simulink model "sampleModel646original"  (R2021b)
settings: Solver=VariableStepAuto  StartTime=0.0  StopTime=10.0  RelTol=1e-3
undefined symbols (not defined in the file): DiscIntNeverNeededParam, Newton, Raphson, sigbuilder_block
libraries: simulink x194, slpidlib x27
(part 5 of 5)

== system sampleModel646original/emi_506 ==
  In1 : Inport
  emi_507 : Inport  Port=2
  emi_509 : Relay
  emi_{510..511,514,519,521,523} (6 alike) : simulink/Discrete/Transfer Fcn First Order  PoleZ=0.95  ICPrevOutput=0.0  DoSatur=off
  emi_512 : Sum  Inputs=+
  emi_513 : DiscreteIntegrator  SampleTime=-1  ICPrevOutput=DiscIntNeverNeededParam  ICPrevScaledInput=DiscIntNeverNeededParam
  emi_515 : DiscreteIntegrator  SampleTime=-1  ICPrevOutput=DiscIntNeverNeededParam  ICPrevScaledInput=DiscIntNeverNeededParam
  emi_516 : DiscreteFir
  emi_517 : Abs
  emi_518 : simulink/Discrete/Difference  ICPrevInput=0.0  OutMin=[]  OutMax=[]  OutDataType=fixdt(1, 16)  OutScaling=2^-10  DoSatur=off
  emi_520 : MinMax
  emi_522 : DiscreteZeroPole  Poles=[0 0.5]  Gain=1  SampleTime=-1
  emi_524 : simulink/Discrete/Discrete Derivative  gainval=1.0  ICPrevScaledInput=0.0  OutMin=[]  OutMax=[]  OutDataType=fixdt(1, 16)  OutScaling=2^-10  DoSatur=off
  emi_525 : simulink/Discrete/Difference  ICPrevInput=0.0  OutMin=[]  OutMax=[]  OutDataType=fixdt(1, 16)  OutScaling=2^-10  DoSatur=off
  emi_526 : Product  Inputs=*
  emi_527 : Math  SaturateOnIntegerOverflow=on
  emi_528 : simulink/Discontinuities/Rate Limiter Dynamic
  emi_529 : Clock
  Out1 : Outport
  emi_508 : Outport  Port=2
  wires:
  In1/1 -> Out1/1
  emi_509/1 -> emi_510/1
  emi_510/1 -> emi_511/1
  emi_511/1 -> emi_512/1
  emi_512/1 -> emi_513/1
  emi_513/1 -> emi_514/1
  emi_514/1 -> emi_515/1
  emi_515/1 -> emi_516/1
  emi_516/1 -> emi_517/1
  emi_517/1 -> emi_518/1
  emi_518/1 -> emi_519/1
  emi_519/1 -> emi_520/1
  emi_520/1 -> emi_521/1
  emi_521/1 -> emi_522/1
  emi_522/1 -> emi_523/1
  emi_523/1 -> emi_524/1
  emi_524/1 -> emi_525/1
  emi_525/1 -> emi_526/1
  emi_526/1 -> emi_527/1
  emi_527/1 -> emi_528/1
  emi_529/1 -> emi_509/1
  emi_528/1 -> emi_508/1

== system sampleModel646original/emi_536 ==
  emi_543 : Inport
  Action Port : ActionPort  ActionPortLabel=if(0 > u1)
  emi_540 : Abs
  emi_{541..542,549..550} (4 alike) : MinMax
  emi_545 : Trigonometry
  emi_546 : Trigonometry
  emi_547 : UnaryMinus
  emi_548 : Sin  TimeSource=Use external signal  SampleTime=0
  emi_551 : Sum  Inputs=+
  emi_552 : Sin  TimeSource=Use external signal  SampleTime=0
  emi_553 : Sqrt  Operator=rSqrt  SaturateOnIntegerOverflow=on
  emi_554 : Ground
  emi_544 : Outport
  wires:
  emi_543/1 -> emi_540/1
  emi_540/1 -> emi_541/1
  emi_541/1 -> emi_542/1
  emi_545/1 -> emi_546/1
  emi_546/1 -> emi_547/1
  emi_547/1 -> emi_548/1
  emi_548/1 -> emi_549/1
  emi_549/1 -> emi_550/1
  emi_550/1 -> emi_551/1
  emi_551/1 -> emi_552/1
  emi_552/1 -> emi_553/1
  emi_554/1 -> emi_545/1
  emi_553/1 -> emi_544/1

== system sampleModel646original/emi_557 ==
  In1 : Inport
  emi_558 : Inport  Port=2
  emi_560 : Gain
  emi_561 : simulink/Discrete/Discrete Derivative  gainval=1.0  ICPrevScaledInput=0.0  OutMin=[]  OutMax=[]  OutDataType=fixdt(1, 16)  OutScaling=2^-10  DoSatur=off
  emi_562 : DiscreteIntegrator  SampleTime=-1  ICPrevOutput=DiscIntNeverNeededParam  ICPrevScaledInput=DiscIntNeverNeededParam
  emi_563 : RateLimiter  SampleTimeMode=inherited
  emi_564 : Product  Inputs=*
  emi_565 : MinMax
  emi_566 : DiscreteTransferFcn
  emi_567 : simulink/Discontinuities/PWM  DisableCoverage=on  Period=1  DisallowZeroDutyCycle=off  RunAtFixedTimeIntervals=off  SampleTime=0.1
  emi_568 : Gain
  emi_569 : Abs
  emi_570 : Trigonometry
  emi_571 : Sqrt  Operator=rSqrt  SaturateOnIntegerOverflow=on
  emi_572 : Sum  Inputs=+
  emi_573 : simulink/Sources/Chirp Signal  f1=0.1  T=100  f2=1
  Out1 : Outport
  emi_559 : Outport  Port=2
  wires:
  In1/1 -> Out1/1
  emi_560/1 -> emi_561/1
  emi_561/1 -> emi_562/1
  emi_562/1 -> emi_563/1
  emi_563/1 -> emi_564/1
  emi_564/1 -> emi_565/1
  emi_565/1 -> emi_566/1
  emi_566/1 -> emi_567/1
  emi_567/1 -> emi_568/1
  emi_568/1 -> emi_569/1
  emi_569/1 -> emi_570/1
  emi_570/1 -> emi_571/1
  emi_571/1 -> emi_572/1
  emi_573/1 -> emi_560/1
  emi_572/1 -> emi_559/1

== system sampleModel646original/emi_580 ==
  emi_587 : Inport
  Action Port : ActionPort  ActionPortLabel=if(0 > u1)
  emi_{584,586,589,594} (4 alike) : Abs
  emi_585 : Math  SaturateOnIntegerOverflow=on
  emi_590 : Gain
  emi_591 : Sqrt  Operator=rSqrt  SaturateOnIntegerOverflow=on
  emi_592 : Gain
  emi_593 : Rounding
  emi_595 : Trigonometry
  emi_596 : Product  Inputs=*
  emi_597 : Sum  Inputs=+
  emi_598 : Rounding
  emi_599 : Sin  TimeSource=Use external signal  SampleTime=0
  emi_600 : Sqrt  Operator=rSqrt  SaturateOnIntegerOverflow=on
  emi_601 : Trigonometry
  emi_602 : Ground
  emi_588 : Outport
  wires:
  emi_587/1 -> emi_584/1
  emi_584/1 -> emi_585/1
  emi_585/1 -> emi_586/1
  emi_589/1 -> emi_590/1
  emi_590/1 -> emi_591/1
  emi_591/1 -> emi_592/1
  emi_592/1 -> emi_593/1
  emi_593/1 -> emi_594/1
  emi_594/1 -> emi_595/1
  emi_595/1 -> emi_596/1
  emi_596/1 -> emi_597/1
  emi_597/1 -> emi_598/1
  emi_598/1 -> emi_599/1
  emi_599/1 -> emi_600/1
  emi_600/1 -> emi_601/1
  emi_602/1 -> emi_589/1
  emi_601/1 -> emi_588/1

== system sampleModel646original/emi_605 ==
  In1 : Inport
  emi_606 : Inport  Port=2
  emi_608 : simulink/Discontinuities/Wrap To Zero  Threshold=255
      settings: SourceProductBaseCode=SL
  emi_609 : simulink/Discontinuities/Rate Limiter Dynamic
  emi_610 : DiscreteTransferFcn
  emi_611 : RateLimiter  SampleTimeMode=inherited
  emi_612 : Gain
  emi_613 : simulink/Discrete/Transfer Fcn First Order  PoleZ=0.95  ICPrevOutput=0.0  DoSatur=off
  emi_614 : simulink/Discontinuities/Saturation Dynamic  OutMin=[]  OutMax=[]  OutDataTypeStr=Inherit: Same as second input  OutDataType=fixdt(1, 16)  OutScaling=2^-10  DoSatur=off
  emi_615 : Sqrt  Operator=rSqrt  SaturateOnIntegerOverflow=on
  emi_616 : Sqrt  Operator=rSqrt  SaturateOnIntegerOverflow=on
  emi_617 : Sin  TimeSource=Use external signal  SampleTime=0
  emi_618 : Clock
  Out1 : Outport
  emi_607 : Outport  Port=2
  wires:
  In1/1 -> Out1/1
  emi_608/1 -> emi_609/1
  emi_609/1 -> emi_610/1
  emi_610/1 -> emi_611/1
  emi_611/1 -> emi_612/1
  emi_612/1 -> emi_613/1
  emi_613/1 -> emi_614/1
  emi_614/1 -> emi_615/1
  emi_615/1 -> emi_616/1
  emi_616/1 -> emi_617/1
  emi_618/1 -> emi_608/1
  emi_617/1 -> emi_607/1

== system sampleModel646original/emi_61 ==
  emi_68 : Inport
  Action Port : ActionPort  ActionPortLabel=if(0 > u1)
  emi_65 : MinMax  SampleTime=1
  emi_66 : MinMax  SampleTime=1
  emi_67 : Math  SampleTime=1  SaturateOnIntegerOverflow=on
  emi_70 : Gain
  emi_71 : UnaryMinus
  emi_72 : Abs
  emi_73 : Gain
  emi_74 : Ground
  emi_69 : Outport
  wires:
  emi_68/1 -> emi_65/1
  emi_65/1 -> emi_66/1
  emi_66/1 -> emi_67/1
  emi_70/1 -> emi_71/1
  emi_71/1 -> emi_72/1
  emi_72/1 -> emi_73/1
  emi_74/1 -> emi_70/1
  emi_73/1 -> emi_69/1

== system sampleModel646original/emi_625 ==
  emi_632 : Inport
  Action Port : ActionPort  ActionPortLabel=if(0 > u1)
  emi_629 : Abs
  emi_{630..631,643,647,649,651} (6 alike) : MinMax
  emi_634 : Product  Inputs=*
  emi_635 : Trigonometry
  emi_636 : Product  Inputs=*
  emi_637 : Sqrt  Operator=rSqrt  SaturateOnIntegerOverflow=on
  emi_638 : UnaryMinus
  emi_639 : Rounding
  emi_640 : Sin  TimeSource=Use external signal  SampleTime=0
  emi_641 : Trigonometry
  emi_642 : Product  Inputs=*
  emi_644 : Trigonometry
  emi_645 : UnaryMinus
  emi_646 : Sin  TimeSource=Use external signal  SampleTime=0
  emi_648 : Gain
  emi_650 : Abs
  emi_652 : Ground
  emi_633 : Outport
  wires:
  emi_632/1 -> emi_629/1
  emi_629/1 -> emi_630/1
  emi_630/1 -> emi_631/1
  emi_634/1 -> emi_635/1
  emi_635/1 -> emi_636/1
  emi_636/1 -> emi_637/1
  emi_637/1 -> emi_638/1
  emi_638/1 -> emi_639/1
  emi_639/1 -> emi_640/1
  emi_640/1 -> emi_641/1
  emi_641/1 -> emi_642/1
  emi_642/1 -> emi_643/1
  emi_643/1 -> emi_644/1
  emi_644/1 -> emi_645/1
  emi_645/1 -> emi_646/1
  emi_646/1 -> emi_647/1
  emi_647/1 -> emi_648/1
  emi_648/1 -> emi_649/1
  emi_649/1 -> emi_650/1
  emi_650/1 -> emi_651/1
  emi_652/1 -> emi_634/1
  emi_651/1 -> emi_633/1

== system sampleModel646original/emi_655 ==
  In1 : Inport
  emi_656 : Inport  Port=2
  emi_658 : Gain
  emi_659 : simulink/Discontinuities/Saturation Dynamic  OutMin=[]  OutMax=[]  OutDataTypeStr=Inherit: Same as second input  OutDataType=fixdt(1, 16)  OutScaling=2^-10  DoSatur=off
  emi_660 : simulink/Discrete/Transfer Fcn First Order  PoleZ=0.95  ICPrevOutput=0.0  DoSatur=off
  emi_661 : Product  Inputs=*
  emi_662 : Relay
  emi_663 : simulink/Discontinuities/Rate Limiter Dynamic
  emi_664 : Sin  TimeSource=Use external signal  SampleTime=0
  emi_665 : DeadZone  SaturateOnIntegerOverflow=on
  emi_666 : DiscreteIntegrator  SampleTime=-1  ICPrevOutput=DiscIntNeverNeededParam  ICPrevScaledInput=DiscIntNeverNeededParam
  emi_667 : Quantizer
  emi_668 : simulink/Discontinuities/Saturation Dynamic  OutMin=[]  OutMax=[]  OutDataTypeStr=Inherit: Same as second input  OutDataType=fixdt(1, 16)  OutScaling=2^-10  DoSatur=off
  emi_669 : UnaryMinus
  emi_670 : VariablePulseGenerator  SampleTime=0.1
  emi_671 : simulink/Discontinuities/Saturation Dynamic  OutMin=[]  OutMax=[]  OutDataTypeStr=Inherit: Same as second input  OutDataType=fixdt(1, 16)  OutScaling=2^-10  DoSatur=off
  emi_672 : simulink/Discrete/Transfer Fcn First Order  PoleZ=0.95  ICPrevOutput=0.0  DoSatur=off
  emi_673 : Abs
  emi_674 : RateLimiter  SampleTimeMode=inherited
  emi_675 : Abs
  emi_676 : Gain
  emi_677 : Rounding
  emi_678 : DiscreteTransferFcn
  emi_679 : VariablePulseGenerator  SampleTime=0.1
  emi_680 : Product  Inputs=*
  emi_681 : simulink/Discontinuities/Wrap To Zero  Threshold=255
      settings: SourceProductBaseCode=SL
  emi_682 : RateLimiter  SampleTimeMode=inherited
  emi_683 : Quantizer
  emi_684 : Relay
  emi_685 : simulink/Discrete/Discrete Derivative  gainval=1.0  ICPrevScaledInput=0.0  OutMin=[]  OutMax=[]  OutDataType=fixdt(1, 16)  OutScaling=2^-10  DoSatur=off
  emi_686 : simulink/Discrete/Transfer Fcn First Order  PoleZ=0.95  ICPrevOutput=0.0  DoSatur=off
  emi_687 : Math  SaturateOnIntegerOverflow=on
  emi_688 : MinMax
  emi_689 : simulink/Sources/Repeating Sequence Interpolated  OutValues=[3 1 4 2 1].'  TimeValues=[0 0.1 0.5 0.6 1].'  LookUpMeth=Interpolation-Use End Values  tsamp=0.01  OutMin=[]  OutMax=[]  OutDataTypeStr=double  OutputDataTypeScalingMode=double  OutDataType=fixdt(0,8)  OutScaling=2^-10
  Out1 : Outport
  emi_657 : Outport  Port=2
  wires:
  In1/1 -> Out1/1
  emi_658/1 -> emi_659/1
  emi_659/1 -> emi_660/1
  emi_660/1 -> emi_661/1
  emi_661/1 -> emi_662/1
  emi_662/1 -> emi_663/1
  emi_663/1 -> emi_664/1
  emi_664/1 -> emi_665/1
  emi_665/1 -> emi_666/1
  emi_666/1 -> emi_667/1
  emi_667/1 -> emi_668/1
  emi_668/1 -> emi_669/1
  emi_669/1 -> emi_670/1
  emi_670/1 -> emi_671/1
  emi_671/1 -> emi_672/1
  emi_672/1 -> emi_673/1
  emi_673/1 -> emi_674/1
  emi_674/1 -> emi_675/1
  emi_675/1 -> emi_676/1
  emi_676/1 -> emi_677/1
  emi_677/1 -> emi_678/1
  emi_678/1 -> emi_679/1
  emi_679/1 -> emi_680/1
  emi_680/1 -> emi_681/1
  emi_681/1 -> emi_682/1
  emi_682/1 -> emi_683/1
  emi_683/1 -> emi_684/1
  emi_684/1 -> emi_685/1
  emi_685/1 -> emi_686/1
  emi_686/1 -> emi_687/1
  emi_687/1 -> emi_688/1
  emi_689/1 -> emi_658/1
  emi_688/1 -> emi_657/1

== system sampleModel646original/emi_697 ==
  emi_704 : Inport
  Action Port : ActionPort  ActionPortLabel=if(0 > u1)
  emi_701 : MinMax
  emi_702 : MinMax
  emi_703 : Gain
  emi_706 : Sin  TimeSource=Use external signal  SampleTime=0
  emi_707 : Trigonometry
  emi_708 : Math  SaturateOnIntegerOverflow=on
  emi_709 : Rounding
  emi_710 : Abs
  emi_711 : MinMax
  emi_712 : Rounding
  emi_713 : Sum  Inputs=+
  emi_714 : Abs
  emi_715 : Ground
  emi_705 : Outport
  wires:
  emi_704/1 -> emi_701/1
  emi_701/1 -> emi_702/1
  emi_702/1 -> emi_703/1
  emi_706/1 -> emi_707/1
  emi_707/1 -> emi_708/1
  emi_708/1 -> emi_709/1
  emi_709/1 -> emi_710/1
  emi_710/1 -> emi_711/1
  emi_711/1 -> emi_712/1
  emi_712/1 -> emi_713/1
  emi_713/1 -> emi_714/1
  emi_715/1 -> emi_706/1
  emi_714/1 -> emi_705/1

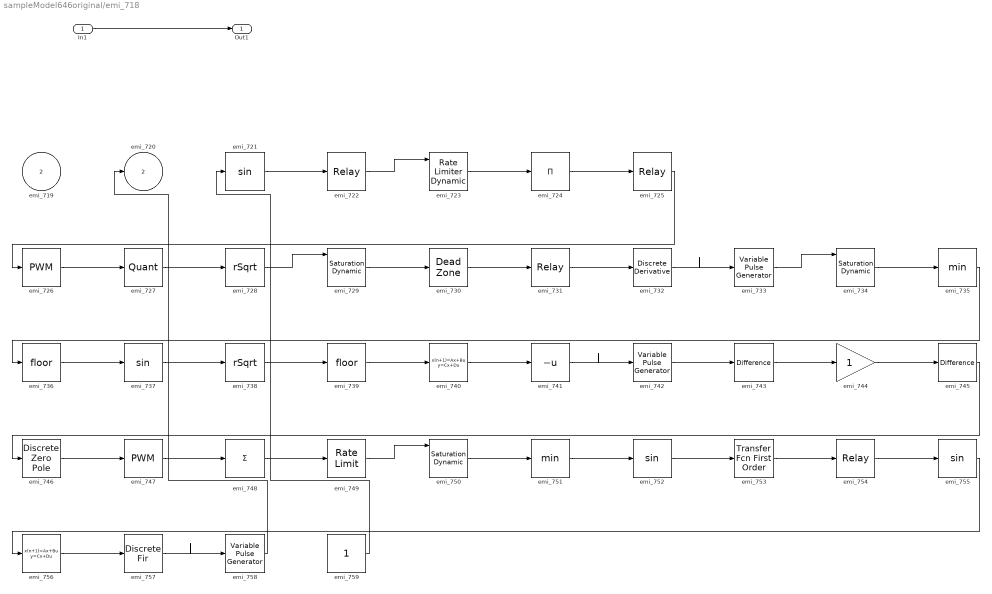
== system sampleModel646original/emi_718 ==
  In1 : Inport
  emi_719 : Inport  Port=2
  emi_{721,737,752,755} (4 alike) : Trigonometry
  emi_{722,725,731,754} (4 alike) : Relay
  emi_723 : simulink/Discontinuities/Rate Limiter Dynamic
  emi_724 : Product  Inputs=*
  emi_726 : simulink/Discontinuities/PWM  DisableCoverage=on  Period=1  DisallowZeroDutyCycle=off  RunAtFixedTimeIntervals=off  SampleTime=0.1
  emi_727 : Quantizer
  emi_728 : Sqrt  Operator=rSqrt  SaturateOnIntegerOverflow=on
  emi_729 : simulink/Discontinuities/Saturation Dynamic  OutMin=[]  OutMax=[]  OutDataTypeStr=Inherit: Same as second input  OutDataType=fixdt(1, 16)  OutScaling=2^-10  DoSatur=off
  emi_730 : DeadZone  SaturateOnIntegerOverflow=on
  emi_732 : simulink/Discrete/Discrete Derivative  gainval=1.0  ICPrevScaledInput=0.0  OutMin=[]  OutMax=[]  OutDataType=fixdt(1, 16)  OutScaling=2^-10  DoSatur=off
  emi_733 : VariablePulseGenerator  SampleTime=0.1
  emi_734 : simulink/Discontinuities/Saturation Dynamic  OutMin=[]  OutMax=[]  OutDataTypeStr=Inherit: Same as second input  OutDataType=fixdt(1, 16)  OutScaling=2^-10  DoSatur=off
  emi_735 : MinMax
  emi_736 : Rounding
  emi_738 : Sqrt  Operator=rSqrt  SaturateOnIntegerOverflow=on
  emi_739 : Rounding
  emi_740 : DiscreteStateSpace  SampleTime=-1
  emi_741 : UnaryMinus
  emi_742 : VariablePulseGenerator  SampleTime=0.1
  emi_743 : simulink/Discrete/Difference  ICPrevInput=0.0  OutMin=[]  OutMax=[]  OutDataType=fixdt(1, 16)  OutScaling=2^-10  DoSatur=off
  emi_744 : Gain
  emi_745 : simulink/Discrete/Difference  ICPrevInput=0.0  OutMin=[]  OutMax=[]  OutDataType=fixdt(1, 16)  OutScaling=2^-10  DoSatur=off
  emi_746 : DiscreteZeroPole  Poles=[0 0.5]  Gain=1  SampleTime=-1
  emi_747 : simulink/Discontinuities/PWM  DisableCoverage=on  Period=1  DisallowZeroDutyCycle=off  RunAtFixedTimeIntervals=off  SampleTime=0.1
  emi_748 : Sum  Inputs=+
  emi_749 : RateLimiter  SampleTimeMode=inherited
  emi_750 : simulink/Discontinuities/Saturation Dynamic  OutMin=[]  OutMax=[]  OutDataTypeStr=Inherit: Same as second input  OutDataType=fixdt(1, 16)  OutScaling=2^-10  DoSatur=off
  emi_751 : MinMax
  emi_753 : simulink/Discrete/Transfer Fcn First Order  PoleZ=0.95  ICPrevOutput=0.0  DoSatur=off
  emi_756 : DiscreteStateSpace  SampleTime=-1
  emi_757 : DiscreteFir
  emi_758 : VariablePulseGenerator  SampleTime=0.1
  emi_759 : Constant
  Out1 : Outport
  emi_720 : Outport  Port=2
  wires:
  In1/1 -> Out1/1
  emi_721/1 -> emi_722/1
  emi_722/1 -> emi_723/1
  emi_723/1 -> emi_724/1
  emi_724/1 -> emi_725/1
  emi_725/1 -> emi_726/1
  emi_726/1 -> emi_727/1
  emi_727/1 -> emi_728/1
  emi_728/1 -> emi_729/1
  emi_729/1 -> emi_730/1
  emi_730/1 -> emi_731/1
  emi_731/1 -> emi_732/1
  emi_732/1 -> emi_733/1
  emi_733/1 -> emi_734/1
  emi_734/1 -> emi_735/1
  emi_735/1 -> emi_736/1
  emi_736/1 -> emi_737/1
  emi_737/1 -> emi_738/1
  emi_738/1 -> emi_739/1
  emi_739/1 -> emi_740/1
  emi_740/1 -> emi_741/1
  emi_741/1 -> emi_742/1
  emi_742/1 -> emi_743/1
  emi_743/1 -> emi_744/1
  emi_744/1 -> emi_745/1
  emi_745/1 -> emi_746/1
  emi_746/1 -> emi_747/1
  emi_747/1 -> emi_748/1
  emi_748/1 -> emi_749/1
  emi_749/1 -> emi_750/1
  emi_750/1 -> emi_751/1
  emi_751/1 -> emi_752/1
  emi_752/1 -> emi_753/1
  emi_753/1 -> emi_754/1
  emi_754/1 -> emi_755/1
  emi_755/1 -> emi_756/1
  emi_756/1 -> emi_757/1
  emi_757/1 -> emi_758/1
  emi_759/1 -> emi_721/1
  emi_758/1 -> emi_720/1

== system sampleModel646original/emi_766 ==
  emi_773 : Inport
  Action Port : ActionPort  ActionPortLabel=if(0 > u1)
  emi_770 : MinMax
  emi_771 : Math  SaturateOnIntegerOverflow=on
  emi_772 : Math  SaturateOnIntegerOverflow=on
  emi_775 : Trigonometry
  emi_776 : Sum  Inputs=+
  emi_777 : Rounding
  emi_778 : Product  Inputs=*
  emi_779 : Trigonometry
  emi_780 : Sin  TimeSource=Use external signal  SampleTime=0
  emi_781 : Abs
  emi_782 : Sqrt  Operator=rSqrt  SaturateOnIntegerOverflow=on
  emi_783 : Sin  TimeSource=Use external signal  SampleTime=0
  emi_784 : Sqrt  Operator=rSqrt  SaturateOnIntegerOverflow=on
  emi_785 : Product  Inputs=*
  emi_786 : MinMax
  emi_787 : Abs
  emi_788 : Abs
  emi_{789,793,795..796} (4 alike) : Gain
  emi_790 : UnaryMinus
  emi_791 : MinMax
  emi_792 : Rounding
  emi_794 : Sqrt  Operator=rSqrt  SaturateOnIntegerOverflow=on
  emi_797 : Ground
  emi_774 : Outport
  wires:
  emi_773/1 -> emi_770/1
  emi_770/1 -> emi_771/1
  emi_771/1 -> emi_772/1
  emi_775/1 -> emi_776/1
  emi_776/1 -> emi_777/1
  emi_777/1 -> emi_778/1
  emi_778/1 -> emi_779/1
  emi_779/1 -> emi_780/1
  emi_780/1 -> emi_781/1
  emi_781/1 -> emi_782/1
  emi_782/1 -> emi_783/1
  emi_783/1 -> emi_784/1
  emi_784/1 -> emi_785/1
  emi_785/1 -> emi_786/1
  emi_786/1 -> emi_787/1
  emi_787/1 -> emi_788/1
  emi_788/1 -> emi_789/1
  emi_789/1 -> emi_790/1
  emi_790/1 -> emi_791/1
  emi_791/1 -> emi_792/1
  emi_792/1 -> emi_793/1
  emi_793/1 -> emi_794/1
  emi_794/1 -> emi_795/1
  emi_795/1 -> emi_796/1
  emi_797/1 -> emi_775/1
  emi_796/1 -> emi_774/1

== system sampleModel646original/emi_77 ==
  In1 : Inport
  emi_78 : Inport  Port=2
  emi_80 : DiscreteIntegrator  SampleTime=-1  ICPrevOutput=DiscIntNeverNeededParam  ICPrevScaledInput=DiscIntNeverNeededParam
  emi_81 : simulink/Discontinuities/Wrap To Zero  Threshold=255
      settings: SourceProductBaseCode=SL
  emi_82 : DigitalClock
  Out1 : Outport
  emi_79 : Outport  Port=2
  wires:
  In1/1 -> Out1/1
  emi_80/1 -> emi_81/1
  emi_82/1 -> emi_80/1
  emi_81/1 -> emi_79/1

== system sampleModel646original/emi_800 ==
  In1 : Inport
  emi_801 : Inport  Port=2
  emi_803 : simulink/Discrete/Transfer Fcn First Order  PoleZ=0.95  ICPrevOutput=0.0  DoSatur=off
  emi_804 : DiscreteFilter
  emi_805 : simulink/Discrete/Transfer Fcn First Order  PoleZ=0.95  ICPrevOutput=0.0  DoSatur=off
  emi_806 : DiscreteZeroPole  Poles=[0 0.5]  Gain=1  SampleTime=-1
  emi_807 : Gain
  emi_808 : DeadZone  SaturateOnIntegerOverflow=on
  emi_809 : simulink/Discrete/Discrete Derivative  gainval=1.0  ICPrevScaledInput=0.0  OutMin=[]  OutMax=[]  OutDataType=fixdt(1, 16)  OutScaling=2^-10  DoSatur=off
  emi_810 : simulink/Discontinuities/PWM  DisableCoverage=on  Period=1  DisallowZeroDutyCycle=off  RunAtFixedTimeIntervals=off  SampleTime=0.1
  emi_{811..813,816,830} (5 alike) : Relay
  emi_814 : DiscreteTransferFcn
  emi_815 : DeadZone  SaturateOnIntegerOverflow=on
  emi_817 : slpidlib/PID Controller  Controller=PID  Form=Parallel  TimeDomain=Discrete-time  UseExternalTs=off  SampleTime=-1  IntegratorMethod=Forward Euler  FilterMethod=Forward Euler  ControllerParametersSource=internal  P=1  I=1  D=0  UseFilter=on  N=100  TunerSelectOption=Transfer Function Based (PID Tuner App)  InitialConditionSource=internal  InitialConditionForIntegrator=0  InitialConditionForFilter=0  DifferentiatorICPrevScaledInput=0  ExternalReset=none  TrackingMode=off  Kt=1  LimitOutput=off  SatLimitsSource=internal  UpperSaturationLimit=inf  LowerSaturationLimit=-inf  LinearizeAsGain=off  AntiWindupMode=none  Kb=1  POutMin=[]  POutMax=[]  IOutMin=[]  IOutMax=[]  DOutMin=[]  DOutMax=[]  NOutMin=[]  NOutMax=[]  SumOutMin=[]  SumOutMax=[]  SaturationOutMin=[]  SaturationOutMax=[]  PParamMin=[]  PParamMax=[]  IParamMin=[]  IParamMax=[]  DParamMin=[]  DParamMax=[]  NParamMin=[]  NParamMax=[]  KbParamMin=[]  KbParamMax=[]  KtParamMin=[]  KtParamMax=[]  KbOutMin=[]  KbOutMax=[]  KtOutMin=[]  KtOutMax=[]  IntegratorOutMin=[]  IntegratorOutMax=[]  FilterOutMin=[]  FilterOutMax=[]  SumI1OutMin=[]  SumI1OutMax=[]  SumI2OutMin=[]  SumI2OutMax=[]  SumI3OutMin=[]  SumI3OutMax=[]  SumI4OutMin=[]  SumI4OutMax=[]  SumDOutMin=[]  SumDOutMax=[]  DifferentiatorOutMin=[]  DifferentiatorOutMax=[]  FilterDiffOutCoefMin=[]  FilterDiffOutCoefMax=[]  ReciprocalOutMin=[]  ReciprocalOutMax=[]  SumDenOutMin=[]  SumDenOutMax=[]  SumNumOutMin=[]  SumNumOutMax=[]  DivideOutMin=[]  DivideOutMax=[]  UdiffTsProdOutMin=[]  UdiffTsProdOutMax=[]  NTsProdOutMin=[]  NTsProdOutMax=[]  UintegralTsProdOutMin=[]  UintegralTsProdOutMax=[]  UngainTsProdOutMin=[]  UngainTsProdOutMax=[]  IntegratorContinuousStateAttributes=''  IntegratorStateMustResolveToSignalObject=off  IntegratorRTWStateStorageClass=Auto  FilterContinuousStateAttributes=''  FilterStateMustResolveToSignalObject=off  FilterRTWStateStorageClass=Auto  ParallelPVariant=InternalParameters  IdealPVariant=Disabled  IVariant=InternalParameters  DVariant=InternalParameters  IntegratorVariant=Discrete  SatVariant=Disabled  AWVariant=Passthrough  PCopyVariant=Disabled  TRVariant=Disabled  FdbkBlocksVariant=Forward  IdealPFdbkVariant=Disabled  SatFdbkVariant=Disabled  DerivativeFilterVariant=ForwardEulerFilter  NVariant=InternalParameters  NCopyVariant=Disabled  FilterICVariant=InternalICsFilter  IntegratorICVariant=InternalICs  ExternalResetVariant=Disabled  TRSumVariant=Passthrough  SumFdbkVariant=Disabled  SumVariant=Sum_PID  TsampFilterVariant=InternalTs  TsampNgainVariant=Passthrough  TsampIntegralVariant=Passthrough  ExternalSaturationOutDataTypeStr=Inherit: Same as second input
  emi_818 : simulink/Discontinuities/Rate Limiter Dynamic
  emi_819 : simulink/Discontinuities/Rate Limiter Dynamic
  emi_820 : DiscreteIntegrator  SampleTime=-1  ICPrevOutput=DiscIntNeverNeededParam  ICPrevScaledInput=DiscIntNeverNeededParam
  emi_821 : Quantizer
  emi_822 : UnaryMinus
  emi_823 : DiscreteIntegrator  SampleTime=-1  ICPrevOutput=DiscIntNeverNeededParam  ICPrevScaledInput=DiscIntNeverNeededParam
  emi_824 : simulink/Discontinuities/PWM  DisableCoverage=on  Period=1  DisallowZeroDutyCycle=off  RunAtFixedTimeIntervals=off  SampleTime=0.1
  emi_825 : simulink/Discontinuities/Saturation Dynamic  OutMin=[]  OutMax=[]  OutDataTypeStr=Inherit: Same as second input  OutDataType=fixdt(1, 16)  OutScaling=2^-10  DoSatur=off
  emi_826 : DiscreteTransferFcn
  emi_827 : Sum  Inputs=+
  emi_828 : Sin  TimeSource=Use external signal  SampleTime=0
  emi_829 : MinMax
  emi_831 : Clock
  Out1 : Outport
  emi_802 : Outport  Port=2
  wires:
  In1/1 -> Out1/1
  emi_803/1 -> emi_804/1
  emi_804/1 -> emi_805/1
  emi_805/1 -> emi_806/1
  emi_806/1 -> emi_807/1
  emi_807/1 -> emi_808/1
  emi_808/1 -> emi_809/1
  emi_809/1 -> emi_810/1
  emi_810/1 -> emi_811/1
  emi_811/1 -> emi_812/1
  emi_812/1 -> emi_813/1
  emi_813/1 -> emi_814/1
  emi_814/1 -> emi_815/1
  emi_815/1 -> emi_816/1
  emi_816/1 -> emi_817/1
  emi_817/1 -> emi_818/1
  emi_818/1 -> emi_819/1
  emi_819/1 -> emi_820/1
  emi_820/1 -> emi_821/1
  emi_821/1 -> emi_822/1
  emi_822/1 -> emi_823/1
  emi_823/1 -> emi_824/1
  emi_824/1 -> emi_825/1
  emi_825/1 -> emi_826/1
  emi_826/1 -> emi_827/1
  emi_827/1 -> emi_828/1
  emi_828/1 -> emi_829/1
  emi_829/1 -> emi_830/1
  emi_831/1 -> emi_803/1
  emi_830/1 -> emi_802/1

== system sampleModel646original/emi_838 ==
  emi_845 : Inport
  Action Port : ActionPort  ActionPortLabel=if(-1.617560e+02 > u1)
  emi_842 : Gain
  emi_843 : Trigonometry
  emi_844 : MinMax
  emi_847 : Gain
  emi_848 : Product  Inputs=*
  emi_849 : Math  SaturateOnIntegerOverflow=on
  emi_850 : Ground
  emi_846 : Outport
  wires:
  emi_845/1 -> emi_842/1
  emi_842/1 -> emi_843/1
  emi_843/1 -> emi_844/1
  emi_847/1 -> emi_848/1
  emi_848/1 -> emi_849/1
  emi_850/1 -> emi_847/1
  emi_849/1 -> emi_846/1

== system sampleModel646original/emi_853 ==
  In1 : Inport
  emi_854 : Inport  Port=2
  emi_856 : slpidlib/PID Controller  Controller=PID  Form=Parallel  TimeDomain=Discrete-time  UseExternalTs=off  SampleTime=-1  IntegratorMethod=Forward Euler  FilterMethod=Forward Euler  ControllerParametersSource=internal  P=1  I=1  D=0  UseFilter=on  N=100  TunerSelectOption=Transfer Function Based (PID Tuner App)  InitialConditionSource=internal  InitialConditionForIntegrator=0  InitialConditionForFilter=0  DifferentiatorICPrevScaledInput=0  ExternalReset=none  TrackingMode=off  Kt=1  LimitOutput=off  SatLimitsSource=internal  UpperSaturationLimit=inf  LowerSaturationLimit=-inf  LinearizeAsGain=off  AntiWindupMode=none  Kb=1  POutMin=[]  POutMax=[]  IOutMin=[]  IOutMax=[]  DOutMin=[]  DOutMax=[]  NOutMin=[]  NOutMax=[]  SumOutMin=[]  SumOutMax=[]  SaturationOutMin=[]  SaturationOutMax=[]  PParamMin=[]  PParamMax=[]  IParamMin=[]  IParamMax=[]  DParamMin=[]  DParamMax=[]  NParamMin=[]  NParamMax=[]  KbParamMin=[]  KbParamMax=[]  KtParamMin=[]  KtParamMax=[]  KbOutMin=[]  KbOutMax=[]  KtOutMin=[]  KtOutMax=[]  IntegratorOutMin=[]  IntegratorOutMax=[]  FilterOutMin=[]  FilterOutMax=[]  SumI1OutMin=[]  SumI1OutMax=[]  SumI2OutMin=[]  SumI2OutMax=[]  SumI3OutMin=[]  SumI3OutMax=[]  SumI4OutMin=[]  SumI4OutMax=[]  SumDOutMin=[]  SumDOutMax=[]  DifferentiatorOutMin=[]  DifferentiatorOutMax=[]  FilterDiffOutCoefMin=[]  FilterDiffOutCoefMax=[]  ReciprocalOutMin=[]  ReciprocalOutMax=[]  SumDenOutMin=[]  SumDenOutMax=[]  SumNumOutMin=[]  SumNumOutMax=[]  DivideOutMin=[]  DivideOutMax=[]  UdiffTsProdOutMin=[]  UdiffTsProdOutMax=[]  NTsProdOutMin=[]  NTsProdOutMax=[]  UintegralTsProdOutMin=[]  UintegralTsProdOutMax=[]  UngainTsProdOutMin=[]  UngainTsProdOutMax=[]  IntegratorContinuousStateAttributes=''  IntegratorStateMustResolveToSignalObject=off  IntegratorRTWStateStorageClass=Auto  FilterContinuousStateAttributes=''  FilterStateMustResolveToSignalObject=off  FilterRTWStateStorageClass=Auto  ParallelPVariant=InternalParameters  IdealPVariant=Disabled  IVariant=InternalParameters  DVariant=InternalParameters  IntegratorVariant=Discrete  SatVariant=Disabled  AWVariant=Passthrough  PCopyVariant=Disabled  TRVariant=Disabled  FdbkBlocksVariant=Forward  IdealPFdbkVariant=Disabled  SatFdbkVariant=Disabled  DerivativeFilterVariant=ForwardEulerFilter  NVariant=InternalParameters  NCopyVariant=Disabled  FilterICVariant=InternalICsFilter  IntegratorICVariant=InternalICs  ExternalResetVariant=Disabled  TRSumVariant=Passthrough  SumFdbkVariant=Disabled  SumVariant=Sum_PID  TsampFilterVariant=InternalTs  TsampNgainVariant=Passthrough  TsampIntegralVariant=Passthrough  ExternalSaturationOutDataTypeStr=Inherit: Same as second input
  emi_857 : DiscreteStateSpace  SampleTime=-1
  emi_858 : Relay
  emi_859 : simulink/Discontinuities/Saturation Dynamic  OutMin=[]  OutMax=[]  OutDataTypeStr=Inherit: Same as second input  OutDataType=fixdt(1, 16)  OutScaling=2^-10  DoSatur=off
  emi_860 : simulink/Discrete/Transfer Fcn First Order  PoleZ=0.95  ICPrevOutput=0.0  DoSatur=off
  emi_861 : DiscreteZeroPole  Poles=[0 0.5]  Gain=1  SampleTime=-1
  emi_862 : Rounding
  emi_863 : Math  SaturateOnIntegerOverflow=on
  emi_864 : Trigonometry
  emi_865 : Sin  TimeSource=Use external signal  SampleTime=0
  emi_866 : simulink/Discrete/Difference  ICPrevInput=0.0  OutMin=[]  OutMax=[]  OutDataType=fixdt(1, 16)  OutScaling=2^-10  DoSatur=off
  emi_867 : DiscreteIntegrator  SampleTime=-1  ICPrevOutput=DiscIntNeverNeededParam  ICPrevScaledInput=DiscIntNeverNeededParam
  emi_868 : DiscreteIntegrator  SampleTime=-1  ICPrevOutput=DiscIntNeverNeededParam  ICPrevScaledInput=DiscIntNeverNeededParam
  emi_869 : Trigonometry
  emi_870 : MinMax
  emi_871 : Sum  Inputs=+
  emi_872 : DiscreteIntegrator  SampleTime=-1  ICPrevOutput=DiscIntNeverNeededParam  ICPrevScaledInput=DiscIntNeverNeededParam
  emi_873 : Rounding
  emi_874 : slpidlib/PID Controller  Controller=PID  Form=Parallel  TimeDomain=Discrete-time  UseExternalTs=off  SampleTime=-1  IntegratorMethod=Forward Euler  FilterMethod=Forward Euler  ControllerParametersSource=internal  P=1  I=1  D=0  UseFilter=on  N=100  TunerSelectOption=Transfer Function Based (PID Tuner App)  InitialConditionSource=internal  InitialConditionForIntegrator=0  InitialConditionForFilter=0  DifferentiatorICPrevScaledInput=0  ExternalReset=none  TrackingMode=off  Kt=1  LimitOutput=off  SatLimitsSource=internal  UpperSaturationLimit=inf  LowerSaturationLimit=-inf  LinearizeAsGain=off  AntiWindupMode=none  Kb=1  POutMin=[]  POutMax=[]  IOutMin=[]  IOutMax=[]  DOutMin=[]  DOutMax=[]  NOutMin=[]  NOutMax=[]  SumOutMin=[]  SumOutMax=[]  SaturationOutMin=[]  SaturationOutMax=[]  PParamMin=[]  PParamMax=[]  IParamMin=[]  IParamMax=[]  DParamMin=[]  DParamMax=[]  NParamMin=[]  NParamMax=[]  KbParamMin=[]  KbParamMax=[]  KtParamMin=[]  KtParamMax=[]  KbOutMin=[]  KbOutMax=[]  KtOutMin=[]  KtOutMax=[]  IntegratorOutMin=[]  IntegratorOutMax=[]  FilterOutMin=[]  FilterOutMax=[]  SumI1OutMin=[]  SumI1OutMax=[]  SumI2OutMin=[]  SumI2OutMax=[]  SumI3OutMin=[]  SumI3OutMax=[]  SumI4OutMin=[]  SumI4OutMax=[]  SumDOutMin=[]  SumDOutMax=[]  DifferentiatorOutMin=[]  DifferentiatorOutMax=[]  FilterDiffOutCoefMin=[]  FilterDiffOutCoefMax=[]  ReciprocalOutMin=[]  ReciprocalOutMax=[]  SumDenOutMin=[]  SumDenOutMax=[]  SumNumOutMin=[]  SumNumOutMax=[]  DivideOutMin=[]  DivideOutMax=[]  UdiffTsProdOutMin=[]  UdiffTsProdOutMax=[]  NTsProdOutMin=[]  NTsProdOutMax=[]  UintegralTsProdOutMin=[]  UintegralTsProdOutMax=[]  UngainTsProdOutMin=[]  UngainTsProdOutMax=[]  IntegratorContinuousStateAttributes=''  IntegratorStateMustResolveToSignalObject=off  IntegratorRTWStateStorageClass=Auto  FilterContinuousStateAttributes=''  FilterStateMustResolveToSignalObject=off  FilterRTWStateStorageClass=Auto  ParallelPVariant=InternalParameters  IdealPVariant=Disabled  IVariant=InternalParameters  DVariant=InternalParameters  IntegratorVariant=Discrete  SatVariant=Disabled  AWVariant=Passthrough  PCopyVariant=Disabled  TRVariant=Disabled  FdbkBlocksVariant=Forward  IdealPFdbkVariant=Disabled  SatFdbkVariant=Disabled  DerivativeFilterVariant=ForwardEulerFilter  NVariant=InternalParameters  NCopyVariant=Disabled  FilterICVariant=InternalICsFilter  IntegratorICVariant=InternalICs  ExternalResetVariant=Disabled  TRSumVariant=Passthrough  SumFdbkVariant=Disabled  SumVariant=Sum_PID  TsampFilterVariant=InternalTs  TsampNgainVariant=Passthrough  TsampIntegralVariant=Passthrough  ExternalSaturationOutDataTypeStr=Inherit: Same as second input
  emi_875 : DiscreteFir
  emi_876 : simulink/Discontinuities/PWM  DisableCoverage=on  Period=1  DisallowZeroDutyCycle=off  RunAtFixedTimeIntervals=off  SampleTime=0.1
  emi_877 : Math  SaturateOnIntegerOverflow=on
  emi_878 : simulink/Discontinuities/Wrap To Zero  Threshold=255
      settings: SourceProductBaseCode=SL
  emi_879 : simulink/Discontinuities/Saturation Dynamic  OutMin=[]  OutMax=[]  OutDataTypeStr=Inherit: Same as second input  OutDataType=fixdt(1, 16)  OutScaling=2^-10  DoSatur=off
  emi_880 : DiscretePulseGenerator  PulseType=Time based  Period=10  PulseWidth=5
  Out1 : Outport
  emi_855 : Outport  Port=2
  wires:
  In1/1 -> Out1/1
  emi_856/1 -> emi_857/1
  emi_857/1 -> emi_858/1
  emi_858/1 -> emi_859/1
  emi_859/1 -> emi_860/1
  emi_860/1 -> emi_861/1
  emi_861/1 -> emi_862/1
  emi_862/1 -> emi_863/1
  emi_863/1 -> emi_864/1
  emi_864/1 -> emi_865/1
  emi_865/1 -> emi_866/1
  emi_866/1 -> emi_867/1
  emi_867/1 -> emi_868/1
  emi_868/1 -> emi_869/1
  emi_869/1 -> emi_870/1
  emi_870/1 -> emi_871/1
  emi_871/1 -> emi_872/1
  emi_872/1 -> emi_873/1
  emi_873/1 -> emi_874/1
  emi_874/1 -> emi_875/1
  emi_875/1 -> emi_876/1
  emi_876/1 -> emi_877/1
  emi_877/1 -> emi_878/1
  emi_878/1 -> emi_879/1
  emi_880/1 -> emi_856/1
  emi_879/1 -> emi_855/1

== system sampleModel646original/emi_888 ==
  emi_895 : Inport
  Action Port : ActionPort  ActionPortLabel=if(0 > u1)
  emi_892 : Math  SaturateOnIntegerOverflow=on
  emi_893 : Trigonometry
  emi_894 : Gain
  emi_897 : Gain
  emi_898 : Gain
  emi_899 : UnaryMinus
  emi_900 : Ground
  emi_896 : Outport
  wires:
  emi_895/1 -> emi_892/1
  emi_892/1 -> emi_893/1
  emi_893/1 -> emi_894/1
  emi_897/1 -> emi_898/1
  emi_898/1 -> emi_899/1
  emi_900/1 -> emi_897/1
  emi_899/1 -> emi_896/1

== system sampleModel646original/emi_89 ==
  emi_96 : Inport
  Action Port : ActionPort  ActionPortLabel=if(0 > u1)
  emi_{100,102,118,121..122,128} (6 alike) : Rounding
  emi_101 : Math  SaturateOnIntegerOverflow=on
  emi_103 : Sum  Inputs=+
  emi_104 : Abs
  emi_105 : Sum  Inputs=+
  emi_106 : Gain
  emi_{107,112,114,116..117} (5 alike) : Sqrt  Operator=rSqrt  SaturateOnIntegerOverflow=on
  emi_108 : MinMax
  emi_109 : UnaryMinus
  emi_110 : UnaryMinus
  emi_111 : Math  SaturateOnIntegerOverflow=on
  emi_113 : Trigonometry
  emi_115 : Sin  TimeSource=Use external signal  SampleTime=0
  emi_119 : Sum  Inputs=+
  emi_120 : Gain
  emi_123 : Product  Inputs=*
  emi_124 : Math  SaturateOnIntegerOverflow=on
  emi_125 : Sin  TimeSource=Use external signal  SampleTime=0
  emi_126 : UnaryMinus
  emi_127 : Sin  TimeSource=Use external signal  SampleTime=0
  emi_129 : Ground
  emi_93 : Abs  SampleTime=1
  emi_94 : MinMax  SampleTime=1
  emi_95 : Gain  SampleTime=1
  emi_98 : Product  Inputs=*
  emi_99 : Abs
  emi_97 : Outport
  wires:
  emi_96/1 -> emi_93/1
  emi_93/1 -> emi_94/1
  emi_94/1 -> emi_95/1
  emi_98/1 -> emi_99/1
  emi_99/1 -> emi_100/1
  emi_100/1 -> emi_101/1
  emi_101/1 -> emi_102/1
  emi_102/1 -> emi_103/1
  emi_103/1 -> emi_104/1
  emi_104/1 -> emi_105/1
  emi_105/1 -> emi_106/1
  emi_106/1 -> emi_107/1
  emi_107/1 -> emi_108/1
  emi_108/1 -> emi_109/1
  emi_109/1 -> emi_110/1
  emi_110/1 -> emi_111/1
  emi_111/1 -> emi_112/1
  emi_112/1 -> emi_113/1
  emi_113/1 -> emi_114/1
  emi_114/1 -> emi_115/1
  emi_115/1 -> emi_116/1
  emi_116/1 -> emi_117/1
  emi_117/1 -> emi_118/1
  emi_118/1 -> emi_119/1
  emi_119/1 -> emi_120/1
  emi_120/1 -> emi_121/1
  emi_121/1 -> emi_122/1
  emi_122/1 -> emi_123/1
  emi_123/1 -> emi_124/1
  emi_124/1 -> emi_125/1
  emi_125/1 -> emi_126/1
  emi_126/1 -> emi_127/1
  emi_127/1 -> emi_128/1
  emi_129/1 -> emi_98/1
  emi_128/1 -> emi_97/1

== system sampleModel646original/emi_903 ==
  In1 : Inport
  emi_904 : Inport  Port=2
  emi_906 : Trigonometry
  emi_907 : DiscreteZeroPole  Poles=[0 0.5]  Gain=1  SampleTime=-1
  emi_908 : simulink/Discrete/Discrete Derivative  gainval=1.0  ICPrevScaledInput=0.0  OutMin=[]  OutMax=[]  OutDataType=fixdt(1, 16)  OutScaling=2^-10  DoSatur=off
  emi_909 : DiscreteFilter
  emi_910 : Rounding
  emi_911 : DiscretePulseGenerator  PulseType=Time based  Period=10  PulseWidth=5
  Out1 : Outport
  emi_905 : Outport  Port=2
  wires:
  In1/1 -> Out1/1
  emi_906/1 -> emi_907/1
  emi_907/1 -> emi_908/1
  emi_908/1 -> emi_909/1
  emi_909/1 -> emi_910/1
  emi_911/1 -> emi_906/1
  emi_910/1 -> emi_905/1

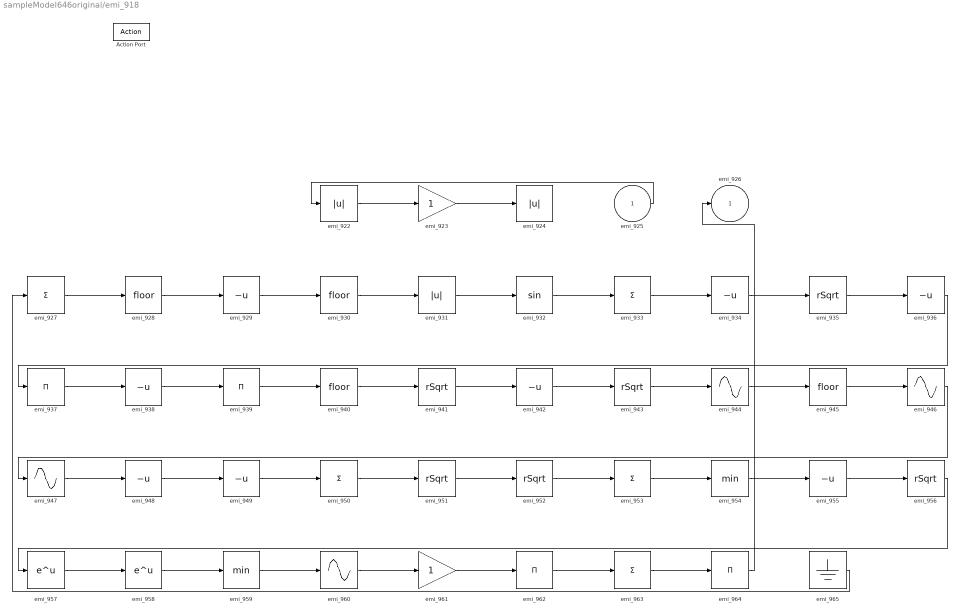
== system sampleModel646original/emi_918 ==
  emi_925 : Inport
  Action Port : ActionPort  ActionPortLabel=if(0 > u1)
  emi_922 : Abs
  emi_923 : Gain
  emi_924 : Abs
  emi_{927,933,950,953,963} (5 alike) : Sum  Inputs=+
  emi_{928,930,940,945} (4 alike) : Rounding
  emi_{929,934,936,938,942,948..949,955} (8 alike) : UnaryMinus
  emi_931 : Abs
  emi_932 : Trigonometry
  emi_{935,941,943,951..952,956} (6 alike) : Sqrt  Operator=rSqrt  SaturateOnIntegerOverflow=on
  emi_{937,939,962,964} (4 alike) : Product  Inputs=*
  emi_{944,946..947,960} (4 alike) : Sin  TimeSource=Use external signal  SampleTime=0
  emi_954 : MinMax
  emi_957 : Math  SaturateOnIntegerOverflow=on
  emi_958 : Math  SaturateOnIntegerOverflow=on
  emi_959 : MinMax
  emi_961 : Gain
  emi_965 : Ground
  emi_926 : Outport
  wires:
  emi_925/1 -> emi_922/1
  emi_922/1 -> emi_923/1
  emi_923/1 -> emi_924/1
  emi_927/1 -> emi_928/1
  emi_928/1 -> emi_929/1
  emi_929/1 -> emi_930/1
  emi_930/1 -> emi_931/1
  emi_931/1 -> emi_932/1
  emi_932/1 -> emi_933/1
  emi_933/1 -> emi_934/1
  emi_934/1 -> emi_935/1
  emi_935/1 -> emi_936/1
  emi_936/1 -> emi_937/1
  emi_937/1 -> emi_938/1
  emi_938/1 -> emi_939/1
  emi_939/1 -> emi_940/1
  emi_940/1 -> emi_941/1
  emi_941/1 -> emi_942/1
  emi_942/1 -> emi_943/1
  emi_943/1 -> emi_944/1
  emi_944/1 -> emi_945/1
  emi_945/1 -> emi_946/1
  emi_946/1 -> emi_947/1
  emi_947/1 -> emi_948/1
  emi_948/1 -> emi_949/1
  emi_949/1 -> emi_950/1
  emi_950/1 -> emi_951/1
  emi_951/1 -> emi_952/1
  emi_952/1 -> emi_953/1
  emi_953/1 -> emi_954/1
  emi_954/1 -> emi_955/1
  emi_955/1 -> emi_956/1
  emi_956/1 -> emi_957/1
  emi_957/1 -> emi_958/1
  emi_958/1 -> emi_959/1
  emi_959/1 -> emi_960/1
  emi_960/1 -> emi_961/1
  emi_961/1 -> emi_962/1
  emi_962/1 -> emi_963/1
  emi_963/1 -> emi_964/1
  emi_965/1 -> emi_927/1
  emi_964/1 -> emi_926/1

== system sampleModel646original/emi_968 ==
  In1 : Inport
  emi_969 : Inport  Port=2
  emi_971 : Math  SaturateOnIntegerOverflow=on
  emi_972 : simulink/Discrete/Discrete Derivative  gainval=1.0  ICPrevScaledInput=0.0  OutMin=[]  OutMax=[]  OutDataType=fixdt(1, 16)  OutScaling=2^-10  DoSatur=off
  emi_973 : Trigonometry
  emi_974 : Rounding
  emi_975 : simulink/Sources/Ramp  slope=1  start=0  InitialOutput=0
  Out1 : Outport
  emi_970 : Outport  Port=2
  wires:
  In1/1 -> Out1/1
  emi_971/1 -> emi_972/1
  emi_972/1 -> emi_973/1
  emi_973/1 -> emi_974/1
  emi_975/1 -> emi_971/1
  emi_974/1 -> emi_970/1

== system sampleModel646original/emi_982 ==
  emi_989 : Inport
  Action Port : ActionPort  ActionPortLabel=if(0 > u1)
  emi_{997,1000,1004,1006..1007} (5 alike) : Sum  Inputs=+
  emi_1001 : Sqrt  Operator=rSqrt  SaturateOnIntegerOverflow=on
  emi_1002 : UnaryMinus
  emi_1003 : Sqrt  Operator=rSqrt  SaturateOnIntegerOverflow=on
  emi_1005 : Product  Inputs=*
  emi_1008 : Abs
  emi_{986,999,1009,1012..1013} (5 alike) : MinMax
  emi_1010 : Product  Inputs=*
  emi_1011 : Product  Inputs=*
  emi_1014 : Ground
  emi_987 : Gain
  emi_988 : Math  SaturateOnIntegerOverflow=on
  emi_991 : Math  SaturateOnIntegerOverflow=on
  emi_992 : Rounding
  emi_993 : Gain
  emi_994 : Rounding
  emi_995 : UnaryMinus
  emi_996 : Sin  TimeSource=Use external signal  SampleTime=0
  emi_998 : Math  SaturateOnIntegerOverflow=on
  emi_990 : Outport
  wires:
  emi_989/1 -> emi_986/1
  emi_986/1 -> emi_987/1
  emi_987/1 -> emi_988/1
  emi_991/1 -> emi_992/1
  emi_992/1 -> emi_993/1
  emi_993/1 -> emi_994/1
  emi_994/1 -> emi_995/1
  emi_995/1 -> emi_996/1
  emi_996/1 -> emi_997/1
  emi_997/1 -> emi_998/1
  emi_998/1 -> emi_999/1
  emi_999/1 -> emi_1000/1
  emi_1000/1 -> emi_1001/1
  emi_1001/1 -> emi_1002/1
  emi_1002/1 -> emi_1003/1
  emi_1003/1 -> emi_1004/1
  emi_1004/1 -> emi_1005/1
  emi_1005/1 -> emi_1006/1
  emi_1006/1 -> emi_1007/1
  emi_1007/1 -> emi_1008/1
  emi_1008/1 -> emi_1009/1
  emi_1009/1 -> emi_1010/1
  emi_1010/1 -> emi_1011/1
  emi_1011/1 -> emi_1012/1
  emi_1012/1 -> emi_1013/1
  emi_1014/1 -> emi_991/1
  emi_1013/1 -> emi_990/1

== system sampleModel646original/cfblk83/cfblk83 ==
  cfblk1 : Inport
  cfblk3 : Sum  Inputs=+-
  cfblk2 : Outport
  wires:
  cfblk3/1 -> cfblk2/1
  cfblk1/1 -> cfblk3/2, cfblk3/1

== system sampleModel646original/emi_456/emi_461 ==
  Demux : Demux  Tag=STV Demux  Outputs=1
      settings: DisplayOption=none
  FromWs : FromWorkspace  Tag=STV FromWs  VariableName=tuvar
      SigBuilderData=|
      | common.afterFinalStr = 'Extrapolate'
      | common.sampleTime = 0
      | dataSet.timeRange = [0 10]
      | dataSet.name = 'Group 1'
      | sbobj.Groups.Name = 'Group 1'
      | sbobj.Groups.Signals.Name = 'Signal 1'
      | sbobj.Groups.Signals.XData = [0 4 4 6 6 10]
      | sbobj.Groups.Signals.YData = [0 0 1 1 0 0]
  Signal 1 : Outport  Tag=STV Outport
  wires:
  Demux/1 -> Signal 1/1
  FromWs/1 -> Demux/1
